simulink model "siso_id"  (R2022b)
settings: Solver=VariableStepAuto  StartTime=0.0  StopTime=10.0  RelTol=1e-3
libraries: cstblocks x10

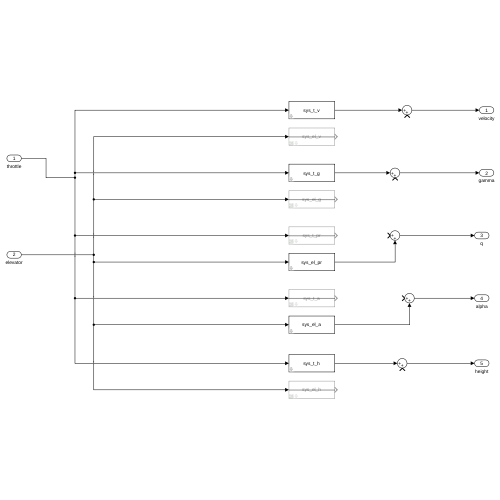
[thumbnail: Simulink's stored preview of the top-level diagram]
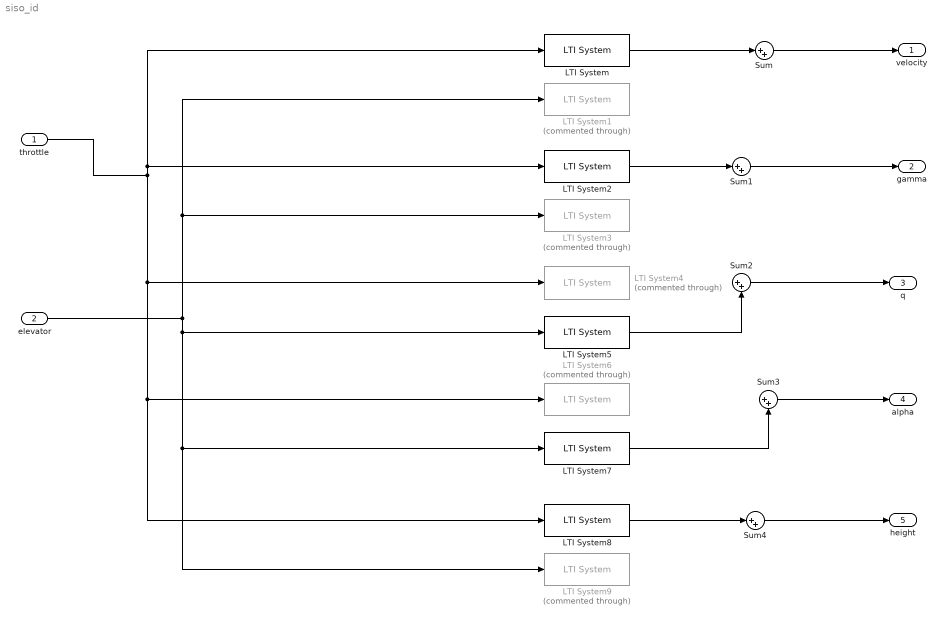
== system siso_id ==
  throttle : Inport
  elevator : Inport  Port=2
  LTI System : cstblocks/LTI System  sys=sys_t_v  IC=[]
  LTI System1 : cstblocks/LTI System  Commented=through  sys=sys_el_v  IC=[]
  LTI System2 : cstblocks/LTI System  sys=sys_t_g  IC=[]
  LTI System3 : cstblocks/LTI System  Commented=through  sys=sys_el_g  IC=[]
  LTI System4 : cstblocks/LTI System  Commented=through  sys=sys_t_pr  IC=[]
  LTI System5 : cstblocks/LTI System  sys=sys_el_pr  IC=[]
  LTI System6 : cstblocks/LTI System  Commented=through  sys=sys_t_a  IC=[]
  LTI System7 : cstblocks/LTI System  sys=sys_el_a  IC=[]
  LTI System8 : cstblocks/LTI System  sys=sys_t_h  IC=[]
  LTI System9 : cstblocks/LTI System  Commented=through  sys=sys_el_h  IC=[]
  Sum{,1..4} (5 alike) : Sum  Inputs=|++
  velocity : Outport
  gamma : Outport  Port=2
  q : Outport  Port=3
  alpha : Outport  Port=4
  height : Outport  Port=5
  wires:
  LTI System/1 -> Sum/1
  Sum/1 -> velocity/1
  LTI System2/1 -> Sum1/1
  Sum1/1 -> gamma/1
  LTI System5/1 -> Sum2/2
  Sum2/1 -> q/1
  LTI System7/1 -> Sum3/2
  Sum3/1 -> alpha/1
  LTI System8/1 -> Sum4/1
  Sum4/1 -> height/1
  throttle/1 -> LTI System2/1, LTI System/1, LTI System4/1, LTI System8/1, LTI System6/1
  elevator/1 -> LTI System3/1, LTI System1/1, LTI System9/1, LTI System7/1, LTI System5/1
